simulink model "SingleLinkManipulator"  (R2021a)
settings: Solver=ode1  StartTime=0.0  StopTime=10.0  RelTol=1e-3
settings Model: Creator=adekoyoa  LastModifiedBy=adekoyoa

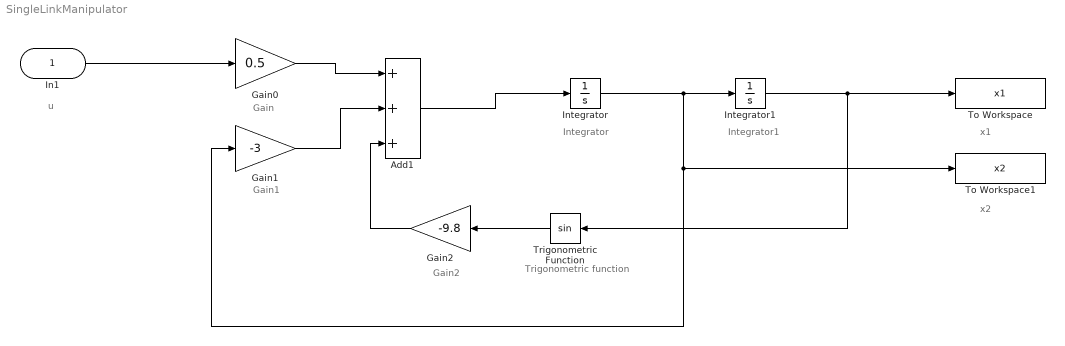
== system SingleLinkManipulator ==
  note: u
  note: Gain2
  note: Trigonometric function
  note: Gain1
  note: Gain
  note: Integrator
  note: Integrator1
  note: x1
  note: x2
  In1 : Inport
  Add1 : Sum  Inputs=+++
  Gain0 : Gain  Gain=0.5
  Gain1 : Gain  Gain=-3
  Gain2 : Gain  Gain=-9.8
  Integrator : Integrator
  Integrator1 : Integrator
  To Workspace : ToWorkspace  VariableName=x1  SampleTime=-1
  To Workspace1 : ToWorkspace  VariableName=x2  SampleTime=-1
  Trigonometric Function : Trigonometry
  wires:
  In1/1 -> Gain0/1
  Gain0/1 -> Add1/1
  Gain1/1 -> Add1/2
  Gain2/1 -> Add1/3
  Add1/1 -> Integrator/1
  Integrator/1 -> To Workspace1/1, Gain1/1, Integrator1/1
  Integrator1/1 -> To Workspace/1, Trigonometric Function/1
  Trigonometric Function/1 -> Gain2/1
